simulink model "cart_pend_part2"  (R2019a)
settings: Solver=FixedStepAuto  StartTime=0.0  StopTime=25  FixedStep=0.001  RelTol=1e-3
values from neighbouring files (symbols this model uses):
  A = Ac    [prepare_sim.m]
  B = [Bc Bwc]    [prepare_sim.m]
  C = eye(4)    [prepare_sim.m]
  D = zeros(4,2)    [prepare_sim.m]
  h = params.h    [prepare_sim.m]
  X0 = [0; 0; 0.1; 0]    [prepare_sim.m]
undefined symbols (not defined in the file or in its folder): dist_enable, tracking_mpc_controller, w
libraries: simulink x1
settings Model: Creator=Piku  LastModifiedBy=laperss

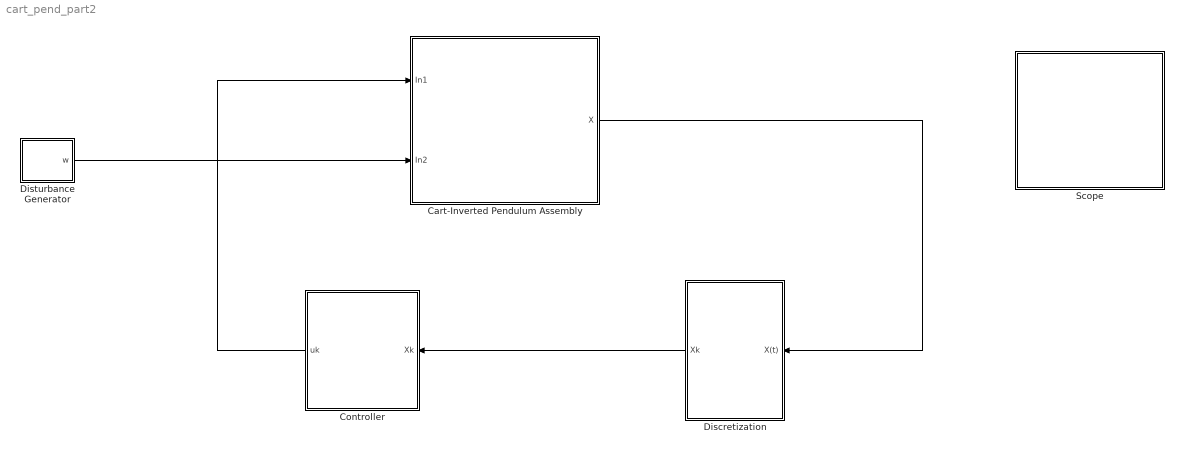
== system cart_pend_part2 ==
  Cart-Inverted Pendulum Assembly : Subsystem
      mask Display: image('cart_pendulum.png');
  Controller : Subsystem
  Discretization : Subsystem
  Disturbance Generator : Subsystem
  Scope : Subsystem
  wires:
  Disturbance Generator/1(w) -> Cart-Inverted Pendulum Assembly/2(In2)
  Controller/1(uk) -> Cart-Inverted Pendulum Assembly/1(In1)
  Cart-Inverted Pendulum Assembly/1("X ") -> Discretization/1(X(t))
  Discretization/1(Xk) -> Controller/1(" Xk")

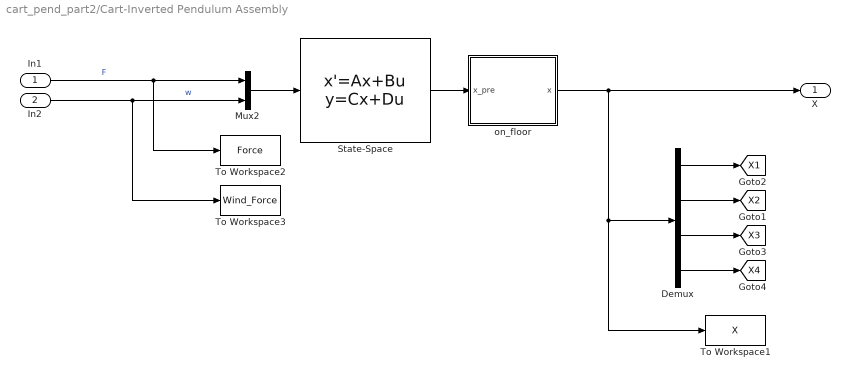
== system cart_pend_part2/Cart-Inverted Pendulum Assembly ==
  In1 : Inport
  In2 : Inport  Port=2
  Demux : Demux
  Mux2 : Mux  Inputs=2
  State-Space : StateSpace  A=A  B=B  C=C  D=D  InitialCondition=X0
  To Workspace1 : ToWorkspace  VariableName=X  SaveFormat=Timeseries  SampleTime=h
  To Workspace2 : ToWorkspace  VariableName=Force  SaveFormat=Timeseries  SampleTime=h
  To Workspace3 : ToWorkspace  VariableName=Wind_Force  SaveFormat=Timeseries  SampleTime=h
  on_floor : Subsystem
  "X " : Outport
  tag scope: X1=global, X2=global, X3=global, X4=global
  wires:
  In1/1 -> Mux2/1, To Workspace2/1  "F"
  State-Space/1 -> on_floor/1(x_pre)
  In2/1 -> To Workspace3/1, Mux2/2  "w"
  Mux2/1 -> State-Space/1
  Demux/1 -> [X1]
  Demux/2 -> [X2]
  Demux/3 -> [X3]
  Demux/4 -> [X4]
  on_floor/1(x) -> To Workspace1/1, Demux/1, "X "/1

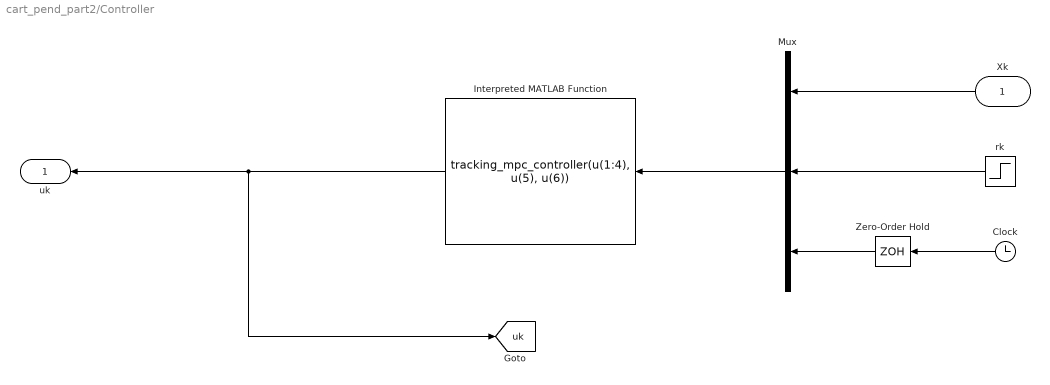
== system cart_pend_part2/Controller ==
  " Xk" : Inport
  Clock : Clock
  Interpreted MATLAB Function : MATLABFcn  MATLABFcn=tracking_mpc_controller(u(1:4), u(5), u(6))  OutputDimensions=1
  Mux : Mux  Inputs=3
  Zero-Order Hold : ZeroOrderHold  SampleTime=h
  rk : Step  Time=0  After=10  SampleTime=h
  uk : Outport
  tag scope: uk=global
  wires:
  " Xk"/1 -> Mux/1
  Interpreted MATLAB Function/1 -> uk/1, [uk]
  Mux/1 -> Interpreted MATLAB Function/1
  Clock/1 -> Zero-Order Hold/1
  Zero-Order Hold/1 -> Mux/3
  rk/1 -> Mux/2

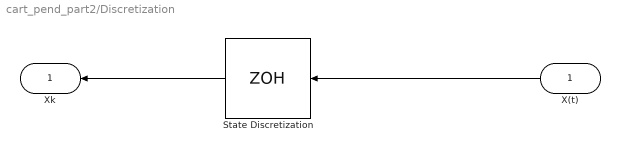
== system cart_pend_part2/Discretization ==
  X(t) : Inport
  State Discretization : ZeroOrderHold  SampleTime=h
  Xk : Outport
  wires:
  X(t)/1 -> State Discretization/1
  State Discretization/1 -> Xk/1

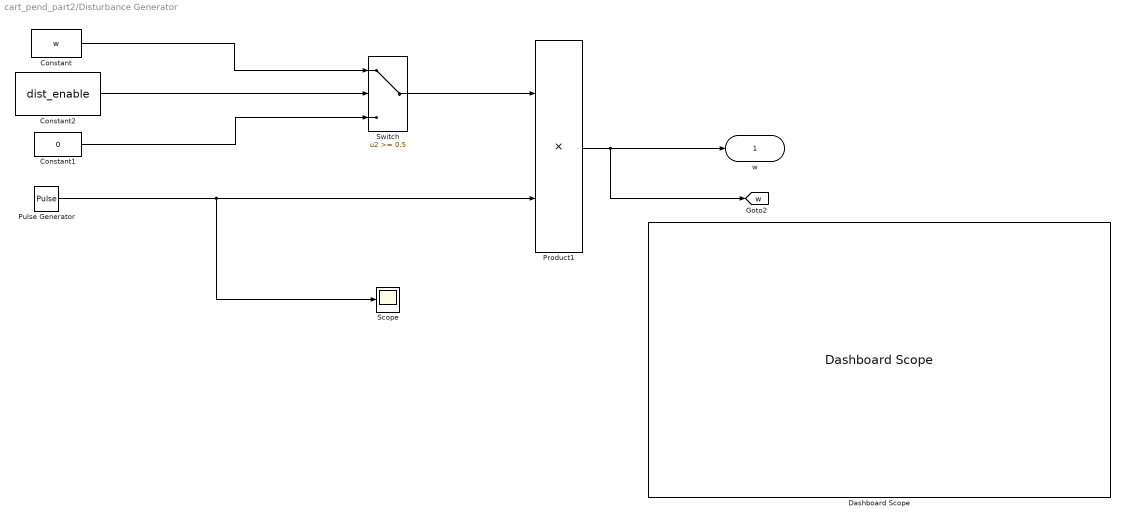
== system cart_pend_part2/Disturbance Generator ==
  Constant : Constant  Value=w
  Constant1 : Constant  Value=0
  Constant2 : Constant  Value=dist_enable
  Dashboard Scope : DashboardScope  Ymin=0  Ymax=0.02
  Product1 : Product
  Pulse Generator : DiscretePulseGenerator  PulseType=Time based  Period=50  PulseWidth=75  PhaseDelay=10
  Scope : Scope
  Switch : Switch  Threshold=0.5
  w : Outport
  tag scope: w=global
  wires:
  Constant2/1 -> Switch/2
  Constant1/1 -> Switch/3
  Constant/1 -> Switch/1
  Switch/1 -> Product1/1
  Product1/1 -> [w], w/1
  Pulse Generator/1 -> Scope/1, Product1/2

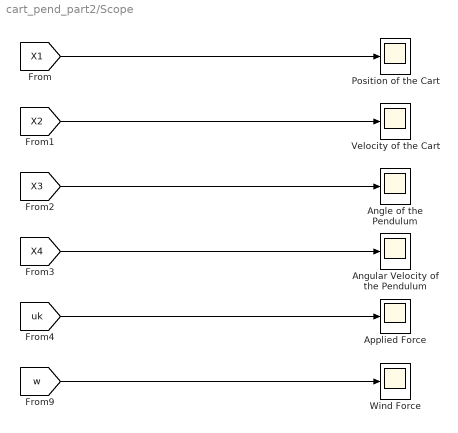
== system cart_pend_part2/Scope ==
  Angle of the Pendulum : Scope
  Angular Velocity of the Pendulum : Scope
  Applied Force : Scope
  Position of the Cart : Scope
  Velocity of the Cart : Scope
  Wind Force : Scope
  wires:
  [uk] -> Applied Force/1
  [X4] -> Angular Velocity of the Pendulum/1
  [X1] -> Position of the Cart/1
  [X2] -> Velocity of the Cart/1
  [X3] -> Angle of the Pendulum/1
  [w] -> Wind Force/1

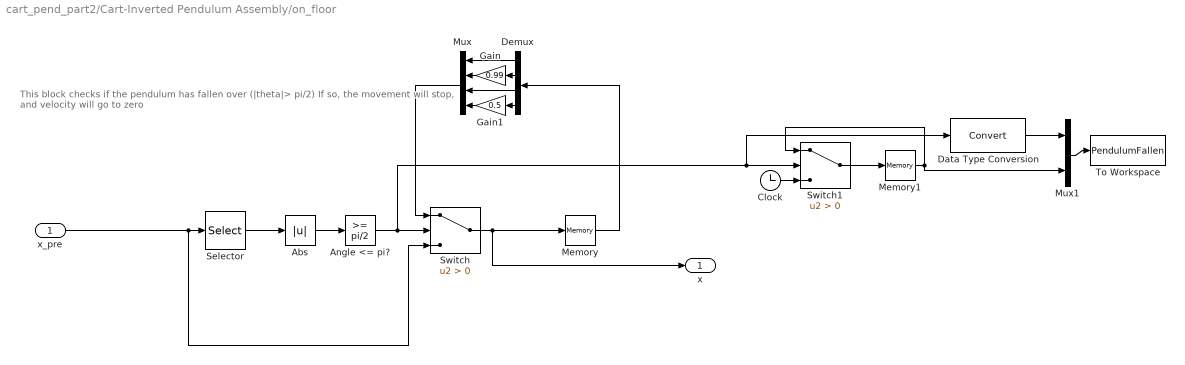
== system cart_pend_part2/Cart-Inverted Pendulum Assembly/on_floor ==
  note: This block checks if the pendulum has fallen over (|theta|> pi/2)
      | If so, the movement will stop, and velocity will go to zero
  x_pre : Inport
  Abs : Abs
  Angle <= pi? : simulink/Logic and Bit Operations/Compare To Constant  relop=>=  const=pi/2  OutDataTypeStr=boolean
  Clock : Clock
  Data Type Conversion : DataTypeConversion
  Demux : Demux
  Gain : Gain  Gain=0.99
  Gain1 : Gain  Gain=0.5
  Memory : Memory
  Memory1 : Memory
  Mux : Mux
  Mux1 : Mux  Inputs=2
  Selector : Selector  InputPortWidth=4  IndexOptions=Index vector (dialog)  Indices=[3]  OutputSizes=1
  Switch : Switch  Criteria=u2 > Threshold
  Switch1 : Switch  Criteria=u2 > Threshold
  To Workspace : ToWorkspace  VariableName=PendulumFallen  SampleTime=-1
      settings: MaxDataPoints=1
  x : Outport
  wires:
  Selector/1 -> Abs/1
  Switch/1 -> x/1, Memory/1
  x_pre/1 -> Switch/3, Selector/1
  Memory/1 -> Demux/1
  Abs/1 -> Angle <= pi?/1
  Demux/1 -> Mux/1
  Demux/3 -> Mux/3
  Gain/1 -> Mux/2
  Demux/2 -> Gain/1
  Demux/4 -> Gain1/1
  Gain1/1 -> Mux/4
  Mux/1 -> Switch/1
  Clock/1 -> Switch1/3
  Switch1/1 -> Memory1/1
  Memory1/1 -> Mux1/2, Switch1/1
  Mux1/1 -> To Workspace/1
  Angle <= pi?/1 -> Data Type Conversion/1, Switch1/2, Switch/2
  Data Type Conversion/1 -> Mux1/1
